simulink model "model_based_imp_ctrl_R2017a"  (Simulink 8.9)
settings: Solver=VariableStepAuto  StartTime=0.0  StopTime=20  FixedStep=0.00040  RelTol=1e-4  AbsTol=1e-7
InitFcn:
  | Parameter
values from neighbouring files (symbols this model uses):
  alpha = pi/180 * 13.6    (= 0.237364778271)    [IdealParameter.m]    (also in ParLuk11.m = deg2rad(13.6); Parameter.m = [-alpha_i;alpha_i;-alpha_i;alpha_i;-alpha_i;alpha_i]; ParameterIdeal.m = [-alpha_i;alpha_i;-alpha_i;alpha_i;-alpha_i;alpha_i]; ParameterVIVE.m = [alpha_i;-alpha_i;alpha_i;-alpha_i;alpha_i;-alpha_i])
  alpha_0 = alpha    (= 0.237364778271)    [IdealParameter.m]    (also in Parameter.m = alpha; ParameterIdeal.m = alpha*1.01; ParameterVIVE.m = alpha*1.01; ParameterVO.m = alpha*1.01)
  angular_noise = 0    [IdealParameter.m]    (also in Parameter.m = 0.5; ParameterIdeal.m; ParameterVIVE.m; ParameterVO.m)
  b = 1.1e-06    [IdealParameter.m]    (also in ParLuk11.m = 1.14e-07; Parameter.m; ParameterIdeal.m; ParameterVIVE.m)
  b_0 = b*1.15    (= 1.265e-06)    [IdealParameter.m]    (also in Parameter.m = 1.1e-06; ParameterIdeal.m; ParameterVIVE.m; ParameterVO.m)
  beta = 0    [IdealParameter.m]    (also in ParLuk11.m; Parameter.m = [beta_i; beta_i; beta_i; beta_i; beta_i; beta_i]; ParameterIdeal.m = [beta_i; beta_i; beta_i; beta_i; beta_i; beta_i]; ParameterVIVE.m = [beta_i; beta_i; beta_i; beta_i; beta_i; beta_i])
  beta_0 = beta    (= 0)    [IdealParameter.m]    (also in Parameter.m = beta; ParameterIdeal.m = beta*0.99; ParameterVIVE.m = beta*0.99; ParameterVO.m = beta*0.99)
  deltah = -0.0427    [Parameter.m]    (also in ParameterIdeal.m; ParameterVIVE.m = 0; ParameterVO.m; Parameter_old.m)
  deltah_0 = deltah    (= -0.0427)    [Parameter.m]    (also in ParameterIdeal.m = -0.041419; ParameterVIVE.m = 0; ParameterVO.m = -0.041419; Parameter_old.m = -0.041419)
  eta_rot = 50    [IdealParameter.m]    (also in Parameter.m = 2; ParameterIdeal.m = 20; ParameterVIVE.m = 5; ParameterVO.m = 2)
  g = 9.81    [IdealParameter.m]    (also in ParLuk11.m; Parameter.m; ParameterIdeal.m; ParameterVIVE.m)
  g_0 = g*0.99    (= 9.7119)    [IdealParameter.m]    (also in Parameter.m = 9.81; ParameterIdeal.m = 9.81; ParameterVIVE.m = 9.81; ParameterVO.m = 9.81)
  IB = [Ixx 0 0; 0 Iyy 0; 0 0 Izz]    [IdealParameter.m]    (also in ParLuk11.m; Parameter.m; ParameterIdeal.m; ParameterVIVE.m)
  IB_0 = IB*1.07    [IdealParameter.m]    (also in Parameter.m = IB; ParameterIdeal.m; ParameterVIVE.m; ParameterVO.m)
  Ip = [Ipx 0 0; 0 Ipy 0; 0 0 Ipz]    [Parameter.m]    (also in ParameterIdeal.m; ParameterVIVE.m; ParameterVO.m; Parameter_old.m)
  k = 5.6e-05    [IdealParameter.m]    (also in ParLuk11.m = 2.98e-06; Parameter.m; ParameterIdeal.m; ParameterVIVE.m = 5.13e-05)
  K_0 = Ts/(T_rotor_0+Ts)    (= 0.0384615384615)    [IdealParameter.m]    (also in Parameter.m = 0.230769230769; ParameterIdeal.m; ParameterVIVE.m = 0.0350877192982; ParameterVO.m = 0.214285714286)
  k_0 = k*1.16    (= 6.496e-05)    [IdealParameter.m]    (also in Parameter.m = 5.6e-05; ParameterIdeal.m; ParameterVIVE.m = 5.9508e-05; ParameterVO.m)
  K_d_star = 4*eye(3)    [Parameter.m]    (also in ParameterIdeal.m; ParameterVIVE.m; ParameterVO.m; Parameter_old.m)
  K_p_star = 50*eye(3)    [Parameter.m]    (also in ParameterIdeal.m; ParameterVIVE.m; ParameterVO.m; Parameter_old.m)
  L = 0.4    [IdealParameter.m]    (also in ParLuk11.m = 1; Parameter.m; ParameterIdeal.m; ParameterVIVE.m = 0.6)
  L_0 = L*1.02    (= 0.408)    [IdealParameter.m]    (also in Parameter.m = 0.4; ParameterIdeal.m; ParameterVIVE.m = 0.612; ParameterVO.m)
  lambda_rot = 10    [IdealParameter.m]    (also in Parameter.m = 3; ParameterIdeal.m; ParameterVIVE.m = 5; ParameterVO.m = 3)
  m = 1    [Controllability.m]    (also in IdealParameter.m = 2.5; ParLuk11.m = 0.6; Parameter.m = 4.85; ParameterIdeal.m = 4.85)
  m_0 = m*1.03    (= 2.575)    [IdealParameter.m]    (also in Parameter.m = 4.85; ParameterIdeal.m = 4.9955; ParameterVIVE.m = 4.52994; ParameterVO.m = 4.9955)
  M_rot = 50    [IdealParameter.m]    (also in Parameter.m = 6; ParameterIdeal.m = 15; ParameterVIVE.m = 1; ParameterVO.m = 6)
  M_star = m_0*eye(3)    [Parameter.m]    (also in ParameterIdeal.m; ParameterVIVE.m; ParameterVO.m; Parameter_old.m)
  mp = 0.05    [Parameter.m]    (also in ParameterIdeal.m; ParameterVIVE.m; ParameterVO.m; Parameter_old.m)
  omega_noise = 0    [IdealParameter.m]    (also in Parameter.m = sqrt(2)*angular_noise/Ts * pi/180; ParameterIdeal.m; ParameterVIVE.m; ParameterVO.m)
  p_noise = 0    [IdealParameter.m]    (also in Parameter.m = 0.001; ParameterIdeal.m; ParameterVIVE.m; ParameterVO.m)
  T_delay = 0    [IdealParameter.m]    (also in Parameter.m = 0.1; ParameterIdeal.m; ParameterVIVE.m = 0.04; ParameterVO.m = 0.1)
  T_rotor = 0.1    [IdealParameter.m]    (also in Parameter.m; ParameterIdeal.m; ParameterVIVE.m; ParameterVO.m)
  Ts = 1/250    (= 0.004)    [IdealParameter.m]    (also in Parameter.m = 0.03; ParameterIdeal.m; ParameterVIVE.m; ParameterVO.m = 0.03)
  v_noise = 0    [IdealParameter.m]    (also in Parameter.m = sqrt(2)*p_noise/Ts; ParameterIdeal.m; ParameterVIVE.m; ParameterVO.m)
  z_p_0 = T_rotor_0/(T_rotor_0+Ts)    (= 0.961538461538)    [IdealParameter.m]    (also in Parameter.m = 0.769230769231; ParameterIdeal.m; ParameterVIVE.m = 0.964912280702; ParameterVO.m = 0.785714285714)
undefined symbols (not defined in the file or in its folder): DiscIntNeverNeededParam, magnitude, mm
libraries: simulink x7, vrlib x2, slctrlblks x1, dspinverses x1
(part 1 of 3)
settings Model: Creator=jan  LastModifiedBy=chao
settings DataIOCC: LimitDataPoints=off  SaveFormat=Dataset  SignalLoggingSaveFormat=Dataset
settings DebuggingCC: UnderspecifiedInitializationDetection=Simplified  MergeDetectMultiDrivingBlocksExec=error  FcnCallInpInsideContextMsg=error  StateNameClashWarn=none  SFUnexpectedBacktrackingDiag=error  SFNoUnconditionalDefaultTransitionDiag=error
settings HardwareCC: ProdBitPerPointer=64  ProdBitPerSizeT=64  ProdBitPerPtrDiffT=64  ProdLargestAtomicFloat=Float  ProdIntDivRoundTo=Zero  ProdEndianess=LittleEndian  ProdWordSize=64  ProdHWDeviceType=Intel->x86-64 (Windows64)
settings ModelReferenceCC: PropagateSignalLabelsOutOfModel=on
settings GRTTargetCC: TargetLangStandard=C99 (ISO)  GeneratePreprocessorConditionals=Use local settings  CombineOutputUpdateFcns=on  GRTInterface=off
settings ConfigComp: CovMetricSettings=dwe  CovHtmlReporting=off  CovSaveCumulativeToWorkspaceVar=off  CovSaveSingleToWorkspaceVar=off  CovExternalEMLEnable=on

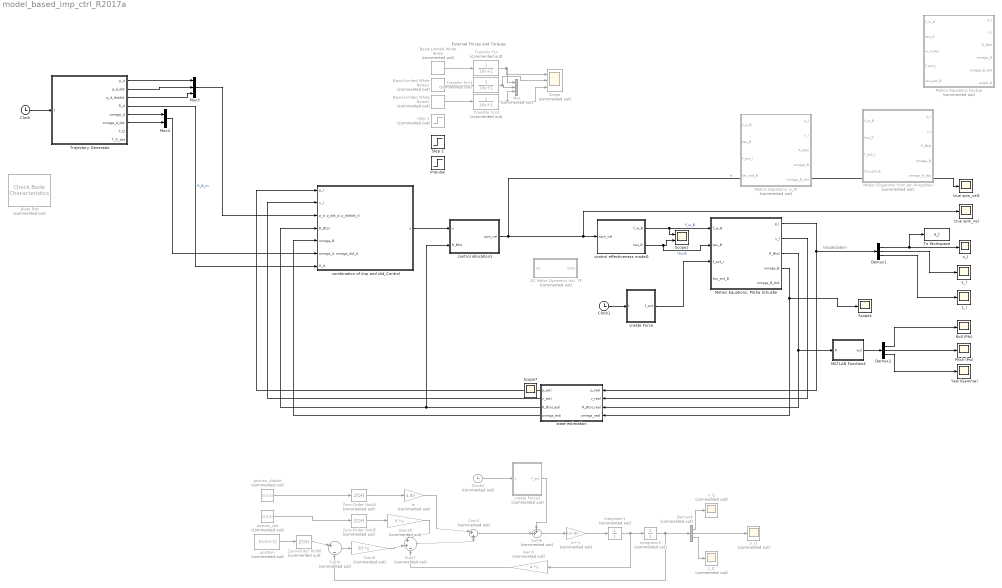
== system model_based_imp_ctrl_R2017a ==
  note: External Forces and Torques
  note: Visualization
  Band-Limited White Noise : simulink/Sources/Band-Limited White Noise  Commented=on  Cov=10  Ts=0.1  seed=[28341]  VectorParams1D=off
  Band-Limited White Noise1 : simulink/Sources/Band-Limited White Noise  Commented=on  Cov=10  Ts=0.1  seed=[23342]  VectorParams1D=off
  Band-Limited White Noise2 : simulink/Sources/Band-Limited White Noise  Commented=on  Cov=10  Ts=0.1  seed=[23441]  VectorParams1D=off
  Bode Plot : slctrlblks/Model Verification/Check Bode  Characteristics  Commented=on  InstantiateOnLoad=on  SaveOperatingPoints=off  LinearizationIOs={'/Trajectory Generator', 1, 'in', 'off', '';'/model3 Integral Sliding Mode Control', 1, 'out', 'off', ''}  LinearizeAt=SnapshotTimes  SnapshotTimes=[0]  TriggerType=rising  SampleTime=auto  RateConversionMethod=zoh  PreWarpFreq=10  UseExactDelayModel=off  UseFullBlockNameLabels=off  UseBusSignalLabels=off  enabled=on  stopWhenAssertionFail=off  export=off  ViewDlgPos=[100.333333333333 199.666666666667 510 390]  OpenViewOnLoad=off  LaunchViewOnOpen=off  FrequencyUnits=rad/s  MagnitudeUnits=dB  PhaseUnits=deg  TimeUnits=seconds  EnableUpperBound=off  UpperBoundFrequencies=[]  UpperBoundMagnitudes=[]  EnableLowerBound=off  LowerBoundFrequencies=[]  LowerBoundMagnitudes=[]
      settings: SourceProductName=Simulink Control Design
  Clock : Clock
  Clock1 : Clock
  Clock4 : Clock  Commented=on
  DC Motor Dynamics incl. FF : Subsystem  Commented=on  TreatAsAtomicUnit=on
  Demux1 : Demux  Outputs=3
  Demux2 : Demux  Outputs=3
  Demux4 : Demux  Commented=on  Outputs=3
  Gain10 : Gain  Commented=on  Gain=4  Multiplication=Matrix(K*u)
  Gain3 : Gain  Commented=on  Gain=4  Multiplication=Matrix(K*u)
  Gain9 : Gain  Commented=on  Gain=50  Multiplication=Matrix(K*u)
  Impulse : Step  Time=0.1  Before=[6,0,6]'  After=[0,0,0]'  SampleTime=0  VectorParams1D=off
  Integrator1 : Integrator  Commented=on  InitialCondition=[0 0 0]'
  Integrator2 : Integrator  Commented=on  InitialCondition=[0 0 0]'
  MATLAB Function4 : MATLAB Function  TreatAsAtomicUnit=on
  Motion Equations backup : Subsystem  Commented=on
  Motion Equations from Jan Krieglstein : Subsystem  Commented=on
  "Motion Equations, Micha Schuster" : Subsystem
  "Motion Equations, p_I3" : Subsystem  Commented=on
  Mux : Mux  Commented=on  Inputs=3
  Mux3 : Mux  Inputs=3
  Mux4 : Mux  Inputs=2
  Pitch (Psi) : Scope
  Roll (Phi) : Scope
  Scope : Scope  Commented=on  NumInputPorts=3
  Scope1 : Scope
  Scope2 : Scope  NumInputPorts=2
  Step 1 : Step  Commented=on  Before=[0;0;0]  After=[10;1;1]  SampleTime=0  VectorParams1D=off
  Step 2 : Step  Before=[0;0;0]  After=[5;1;1]  SampleTime=0  VectorParams1D=off
  Sum3 : Sum  Commented=on  Inputs=|+|+
  Sum6 : Sum  Commented=on  Inputs=++|
  Sum7 : Sum  Commented=on  Inputs=|+|+|-
  Sum8 : Sum  Commented=on  Inputs=|+|-
  To Workspace : ToWorkspace  VariableName=x_I  SaveFormat=Timeseries  SampleTime=-1
  Trajectory Generator : MATLAB Function  TreatAsAtomicUnit=on
  Transfer Fcn : TransferFcn  Commented=on  Denominator=[10 1]
  Transfer Fcn1 : TransferFcn  Commented=on  Denominator=[10 1]
  Transfer Fcn2 : TransferFcn  Commented=on  Denominator=[10 1]
  Yaw (Gamma) : Scope
  Zero-Order Hold4 : ZeroOrderHold  Commented=on  SampleTime=Ts
  Zero-Order Hold5 : ZeroOrderHold  Commented=on  SampleTime=Ts
  Zero-Order Hold6 : ZeroOrderHold  Commented=on  SampleTime=Ts
  combination of Imp and slid_Control : Subsystem
  control allocation1 : Subsystem
  control effectiveness model1 : Subsystem
  create Force : MATLAB Function  TreatAsAtomicUnit=on
  create Force2 : MATLAB Function  Commented=on  TreatAsAtomicUnit=on
  m : Gain  Commented=on  Gain=4.85
  m*-1 : Gain  Commented=on  Gain=1/4.85
  position : Constant  Commented=on  Value=[0;0;0.5]
  postion_dot : Constant  Commented=on  Value=[0;0;0]
  postion_dotdot : Constant  Commented=on  Value=[0;0;0]
  state estimation : Subsystem
  true spin_vel : Scope
  true spin_vel1 : Scope
  x_I : Scope
  x_I1 : Scope  Commented=on
  y_I : Scope
  y_I1 : Scope  Commented=on
  z_I : Scope
  z_I1 : Scope  Commented=on
  Scope7 : Scope
  wires:
  Demux2/2 -> Pitch (Psi)/1
  Demux1/3 -> z_I/1
  control allocation1/1(spin_vel) -> control effectiveness model1/1(spin_vel), true spin_vel/1, true spin_vel1/1  "u"
  Demux1/2 -> y_I/1
  Demux2/1 -> Roll (Phi)/1
  "Motion Equations, Micha Schuster"/3(R_BtoI) -> MATLAB Function4/1(R), state estimation/3(R_BtoI_real)
  Clock/1 -> Trajectory Generator/1(t)
  Trajectory Generator/3(p_d_dotdot) -> Mux3/3
  Trajectory Generator/2(p_d_dot) -> Mux3/2
  Trajectory Generator/6(omega_d_dot) -> Mux4/2
  Band-Limited White Noise/1 -> Transfer Fcn/1
  Transfer Fcn/1 -> Scope/1, Mux/1
  Transfer Fcn2/1 -> Scope/3, Mux/3
  Band-Limited White Noise1/1 -> Transfer Fcn1/1
  Band-Limited White Noise2/1 -> Transfer Fcn2/1
  Transfer Fcn1/1 -> Scope/2, Mux/2
  Trajectory Generator/5(omega_d) -> Mux4/1
  Demux2/3 -> Yaw (Gamma)/1
  MATLAB Function4/1(eul) -> Demux2/1
  "Motion Equations, Micha Schuster"/1(p_I) -> state estimation/1(p_real), Demux1/1
  Trajectory Generator/4(R_d) -> combination of Imp and slid_Control/7(R_d)  "R_B_m"
  Mux3/1 -> combination of Imp and slid_Control/3("p_d, p_dot_d, p_dotdot_d")
  Mux4/1 -> combination of Imp and slid_Control/6("omega_d, omega_dot_d")
  Clock1/1 -> create Force/1(t)
  Trajectory Generator/1(p_d) -> Mux3/1
  Gain10/1 -> Sum7/1
  Zero-Order Hold6/1 -> Sum8/1
  Integrator2/1 -> Demux4/1, Sum8/2
  m*-1/1 -> Integrator1/1
  Demux4/1 -> x_I1/1
  Sum7/1 -> Sum3/2
  postion_dot/1 -> Zero-Order Hold5/1
  Demux4/2 -> y_I1/1
  Zero-Order Hold4/1 -> m/1
  Sum6/1 -> m*-1/1
  Integrator1/1 -> Gain3/1, Integrator2/1
  position/1 -> Zero-Order Hold6/1
  Zero-Order Hold5/1 -> Gain10/1
  m/1 -> Sum3/1
  Sum3/1 -> Sum6/2
  Demux4/3 -> z_I1/1
  Gain9/1 -> Sum7/2
  Gain3/1 -> Sum7/3
  postion_dotdot/1 -> Zero-Order Hold4/1
  Sum8/1 -> Gain9/1
  create Force2/1(f_ext) -> Sum6/1
  Clock4/1 -> create Force2/1(t)
  combination of Imp and slid_Control/1(u) -> control allocation1/1(u)
  state estimation/3(R_BtoI_esti) -> control allocation1/2(R_BtoI), combination of Imp and slid_Control/4(R_BtoI)
  state estimation/4(omega_esti) -> combination of Imp and slid_Control/5(omega_B)
  state estimation/2(v_esti) -> combination of Imp and slid_Control/2(v_I)
  state estimation/1(p_esti) -> combination of Imp and slid_Control/1(p_I)
  "Motion Equations, Micha Schuster"/2(v_I) -> state estimation/2(v_real)
  "Motion Equations, Micha Schuster"/4(omega_B) -> Scope1/1, state estimation/4(omega_real)
  control effectiveness model1/1(f_w_B) -> "Motion Equations, Micha Schuster"/1("f_w_B "), Scope2/1  "f_w_B"
  control effectiveness model1/2(tau_B) -> "Motion Equations, Micha Schuster"/2(tau_B), Scope2/2  "tau_B"
  create Force/1(f_ext) -> "Motion Equations, Micha Schuster"/3(f_ext_I)
  Demux1/1 -> To Workspace/1, x_I/1

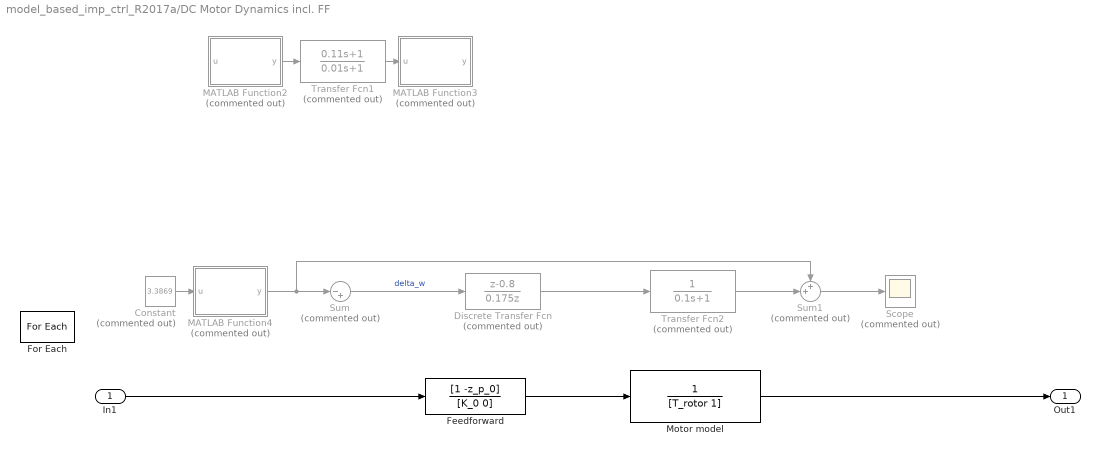
== system model_based_imp_ctrl_R2017a/DC Motor Dynamics incl. FF ==
  In1 : Inport  Partition=on  PartitionDimension=1  PartitionWidth=1
  Constant : Constant  Commented=on  Value=3.3869
  Discrete Transfer Fcn : DiscreteTransferFcn  Commented=on  Numerator=[1 -0.8]  Denominator=[0.175 0]  SampleTime=Ts
  Feedforward : DiscreteTransferFcn  Numerator=[1 -z_p_0]  Denominator=[K_0 0]  InitialStates=274  SampleTime=Ts
  For Each : ForEach  DisableCoverage=on  IndexMode=One-based
  MATLAB Function2 : MATLAB Function  Commented=on  TreatAsAtomicUnit=on
  MATLAB Function3 : MATLAB Function  Commented=on  TreatAsAtomicUnit=on
  MATLAB Function4 : MATLAB Function  Commented=on  TreatAsAtomicUnit=on
  Motor model : TransferFcn  Denominator=[T_rotor 1]
  Scope : Scope  Commented=on
  Sum : Sum  Commented=on  Inputs=|-+
  Sum1 : Sum  Commented=on  Inputs=++|
  Transfer Fcn1 : TransferFcn  Commented=on  Numerator=[0.11 1]  Denominator=[0.01 1]
  Transfer Fcn2 : TransferFcn  Commented=on  Denominator=[0.1 1]
  Out1 : Outport  ConcatenationDimension=1
  wires:
  Transfer Fcn1/1 -> MATLAB Function3/1(u)
  MATLAB Function2/1(y) -> Transfer Fcn1/1
  Constant/1 -> MATLAB Function4/1(u)
  MATLAB Function4/1(y) -> Sum1/1, Sum/1
  Sum/1 -> Discrete Transfer Fcn/1  "delta_w"
  In1/1 -> Feedforward/1
  Discrete Transfer Fcn/1 -> Transfer Fcn2/1
  Transfer Fcn2/1 -> Sum1/2
  Motor model/1 -> Out1/1
  Sum1/1 -> Scope/1
  Feedforward/1 -> Motor model/1

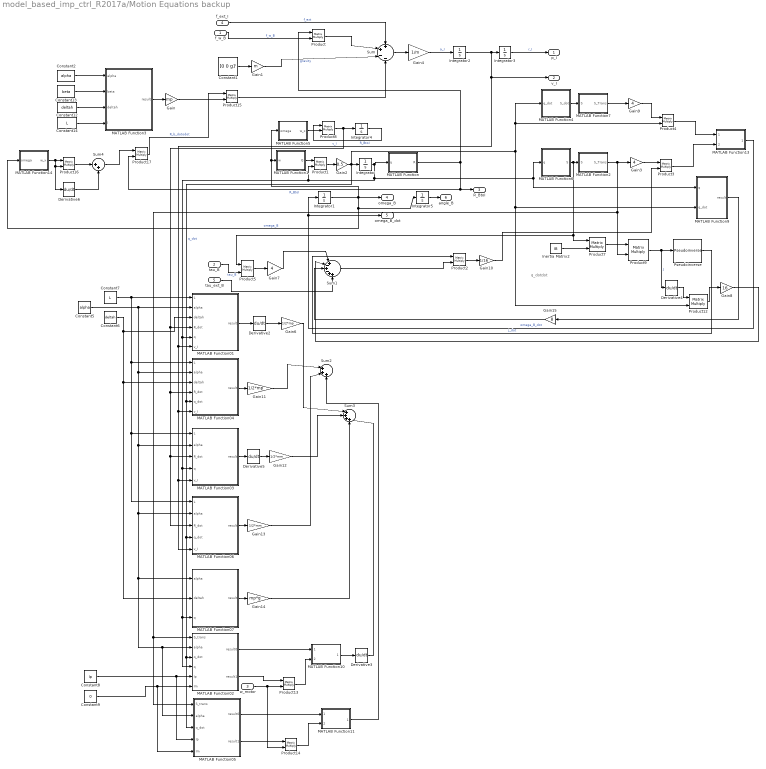
== system model_based_imp_ctrl_R2017a/Motion Equations backup ==
  note: q_dotdot
  "f_w_B " : Inport
  tau_B : Inport  Port=2
  w_motor : Inport  Port=3
  f_ext_I : Inport  Port=4
  tau_ext_B : Inport  Port=5
  Constant1 : Constant  Value=[0 0 g]'  VectorParams1D=off
  Constant12 : Constant  Value=deltah
  Constant13 : Constant  Value=beta
  Constant14 : Constant  Value=L
  Constant2 : Constant  Value=alpha
  Constant5 : Constant  Value=alpha
  Constant6 : Constant  Value=deltah
  Constant7 : Constant  Value=L
  Constant8 : Constant  Value=Ip
  Constant9 : Constant  Value=0
  Derivative{2..6} (5 alike) : Derivative  CoefficientInTFapproximation=0
  Gain : Gain  Gain=mp
  Gain1 : Gain  Gain=m
  Gain10 : Gain  Gain=1/16
  Gain11 : Gain  Gain=1/2*mp
  Gain12 : Gain  Gain=1/2*mm
  Gain13 : Gain  Gain=1/2*mm
  Gain14 : Gain  Gain=mp*g
  Gain15 : Gain  Gain=8
  Gain2 : Gain  Gain=0.5
  Gain3 : Gain  Gain=4
  Gain4 : Gain  Gain=1/m
  Gain6 : Gain  Gain=1/2*mp
  Gain7 : Gain  Gain=4
  Gain8 : Gain  Gain=16
  Gain9 : Gain  Gain=4
  Inertia Matrix2 : Constant  Value=IB  VectorParams1D=off
  Integrator : Integrator  InitialCondition=[0 0 0 1]
  Integrator1 : Integrator  InitialCondition=[0 0 0]'
  Integrator2 : Integrator  InitialCondition=[0;0;0]
  Integrator3 : Integrator  InitialCondition=[0 0 0]'
  Integrator4 : Integrator  InitialCondition=[1 0 0; 0 1 0; 0 0 1]
  Integrator5 : Integrator  InitialCondition=[0 0 0]'
  MATLAB Function : MATLAB Function  TreatAsAtomicUnit=on
  MATLAB Function01 : MATLAB Function  TreatAsAtomicUnit=on
  MATLAB Function02 : MATLAB Function  TreatAsAtomicUnit=on
  MATLAB Function03 : MATLAB Function  TreatAsAtomicUnit=on
  MATLAB Function04 : MATLAB Function  TreatAsAtomicUnit=on
  MATLAB Function05 : MATLAB Function  TreatAsAtomicUnit=on
  MATLAB Function06 : MATLAB Function  TreatAsAtomicUnit=on
  MATLAB Function07 : MATLAB Function  TreatAsAtomicUnit=on
  MATLAB Function1 : MATLAB Function  TreatAsAtomicUnit=on
  MATLAB Function10 : MATLAB Function  TreatAsAtomicUnit=on
  MATLAB Function11 : MATLAB Function  TreatAsAtomicUnit=on
  MATLAB Function13 : MATLAB Function  TreatAsAtomicUnit=on
  MATLAB Function14 : MATLAB Function  TreatAsAtomicUnit=on
  MATLAB Function2 : MATLAB Function  TreatAsAtomicUnit=on
  MATLAB Function3 : MATLAB Function  TreatAsAtomicUnit=on
  MATLAB Function4 : MATLAB Function  TreatAsAtomicUnit=on
  MATLAB Function5 : MATLAB Function  TreatAsAtomicUnit=on
  MATLAB Function6 : MATLAB Function  TreatAsAtomicUnit=on
  MATLAB Function7 : MATLAB Function  TreatAsAtomicUnit=on
  MATLAB Function9 : MATLAB Function  TreatAsAtomicUnit=on
  Product{,1..5,7..9,12..17} (15 alike) : Product  Multiplication=Matrix(*)
  Pseudoinverse : dspinverses/Pseudoinverse  wanterr=off  SimulateUsing=Interpreted execution
      settings: SourceProductName=DSP System Toolbox  SourceProductBaseCode=DS
  Sum : Sum  Inputs=++--
  Sum1 : Sum  Inputs=|+-+-++
  Sum2 : Sum  Inputs=|+++
  Sum3 : Sum  Inputs=|++++
  Sum4 : Sum  Inputs=|++
  p_I : Outport
  v_I : Outport  Port=2
  R_BtoI : Outport  Port=3
  omega_B : Outport  Port=4
  omega_B_dot : Outport  Port=5
  angle_B : Outport  Port=6
  wires:
  Gain4/1 -> Integrator2/1  "a_I"
  Constant1/1 -> Gain1/1
  Gain2/1 -> MATLAB Function04/5(q_dot), MATLAB Function06/4(q_dot), MATLAB Function05/3(q_dot), MATLAB Function02/3(q_dot), MATLAB Function4/1(q_dot), Product4/2, MATLAB Function9/2(q_dot), Product12/2, Integrator/1  "q_dot"
  Integrator2/1 -> MATLAB Function06/5(v_I), MATLAB Function03/5(v_I), MATLAB Function04/6(v_I), MATLAB Function01/6(v_I), v_I/1, Integrator3/1  "v_I"
  Sum/1 -> Gain4/1
  "f_w_B "/1 -> Product/2  "f_w_B"
  Product1/1 -> Gain2/1
  Integrator3/1 -> p_I/1  "r_I"
  MATLAB Function1/1(Q) -> Product1/1
  MATLAB Function/1(R) -> Product/1, Product17/2, R_BtoI/1  "R_BtoI"
  tau_B/1 -> Product5/2  "tau_B"
  Sum1/1 -> Product2/2
  MATLAB Function4/1(S_dot) -> MATLAB Function7/1(S)
  MATLAB Function7/1(S_Trans) -> Gain9/1
  Gain3/1 -> Product3/1
  Gain9/1 -> Product4/1
  Product4/1 -> MATLAB Function13/1(factor1)
  Product3/1 -> MATLAB Function13/2(factor2)
  MATLAB Function13/1(add_result) -> Integrator1/1, omega_B_dot/1  "omega_B_dot"
  MATLAB Function6/1(S) -> Product5/1, Product7/1, MATLAB Function2/1(S)
  Product5/1 -> Gain7/1
  Gain7/1 -> Sum1/1
  Inertia Matrix2/1 -> Product7/2
  Product7/1 -> Product9/1
  Product9/1 -> Derivative4/1, Pseudoinverse/1  "J"
  Pseudoinverse/1 -> Product2/1  "j_dot"
  Derivative4/1 -> Product12/1
  Product8/1 -> MATLAB Function06/3(R_dot), MATLAB Function03/3(R_dot), MATLAB Function04/4(R_dot), MATLAB Function01/4(R_dot), Integrator4/1
  Integrator4/1 -> Product8/1  "R_BtoI"
  MATLAB Function5/1(w_x) -> Product8/2
  Integrator1/1 -> MATLAB Function14/1(omega), Integrator5/1, MATLAB Function5/1(omega), MATLAB Function1/1(w), omega_B/1  "omega_B"
  Derivative2/1 -> Gain6/1
  MATLAB Function01/1(result) -> Derivative2/1
  Constant6/1 -> MATLAB Function07/2(deltah), MATLAB Function04/3(deltah), MATLAB Function01/3(deltah)
  Constant5/1 -> MATLAB Function03/2(alpha), MATLAB Function06/2(alpha), MATLAB Function07/1(alpha), MATLAB Function05/2(alpha), MATLAB Function02/2(alpha), MATLAB Function04/2(alpha), MATLAB Function01/2(alpha)
  Product12/1 -> Gain8/1
  Gain8/1 -> Sum1/2
  Product2/1 -> Gain10/1
  Gain10/1 -> Product3/2
  Integrator/1 -> MATLAB Function03/4(q), MATLAB Function07/3(q), MATLAB Function02/4(q), MATLAB Function01/5(q), Product1/2, MATLAB Function6/1(q), MATLAB Function9/1(q), MATLAB Function/1(q)
  Constant7/1 -> MATLAB Function06/1(L), MATLAB Function03/1(L), MATLAB Function04/1(L), MATLAB Function01/1(L)
  MATLAB Function04/1(result) -> Gain11/1
  MATLAB Function2/1(S_Trans) -> MATLAB Function05/1(S_trans), MATLAB Function02/1(S_trans), Product9/2, Gain3/1
  Constant8/1 -> MATLAB Function05/4(Ip), MATLAB Function02/5(Ip)
  Constant9/1 -> MATLAB Function05/5(Im), MATLAB Function02/6(Im)
  MATLAB Function03/1(result) -> Derivative5/1
  Derivative5/1 -> Gain12/1
  MATLAB Function06/1(result) -> Gain13/1
  MATLAB Function07/1(result) -> Gain14/1
  Gain6/1 -> Sum3/1
  Gain11/1 -> Sum2/1
  Gain12/1 -> Sum3/2
  Gain13/1 -> Sum2/2
  MATLAB Function02/2(result1) -> Product13/1
  MATLAB Function02/1(result0) -> MATLAB Function10/1(factor1)
  Product13/1 -> MATLAB Function10/2(factor2)
  MATLAB Function10/1(add_result) -> Derivative3/1
  Gain14/1 -> Sum3/4
  Derivative3/1 -> Sum3/3
  w_motor/1 -> Product14/2, Product13/2
  MATLAB Function05/2(result1) -> Product14/1
  MATLAB Function05/1(result0) -> MATLAB Function11/1(factor1)
  Product14/1 -> MATLAB Function11/2(factor2)
  MATLAB Function11/1(add_result) -> Sum2/3
  MATLAB Function9/1(result) -> Gain15/1
  Gain15/1 -> Sum1/3
  f_ext_I/1 -> Sum/1  "f_ext"
  Product/1 -> Sum/2
  Gain1/1 -> Sum/3  "gravity"
  tau_ext_B/1 -> Sum1/6
  Integrator5/1 -> angle_B/1
  Product17/1 -> Product15/1  "R_b_dotodot"
  Product15/1 -> Sum/4
  MATLAB Function14/1(w_x) -> Derivative6/1, Product16/2, Product16/1
  Product16/1 -> Sum4/1
  Derivative6/1 -> Sum4/2
  Sum4/1 -> Product17/1
  Constant13/1 -> MATLAB Function3/2(beta)
  Constant2/1 -> MATLAB Function3/1(alpha)
  Constant12/1 -> MATLAB Function3/3(deltah)
  MATLAB Function3/1(result) -> Gain/1
  Constant14/1 -> MATLAB Function3/4(l)
  Gain/1 -> Product15/2

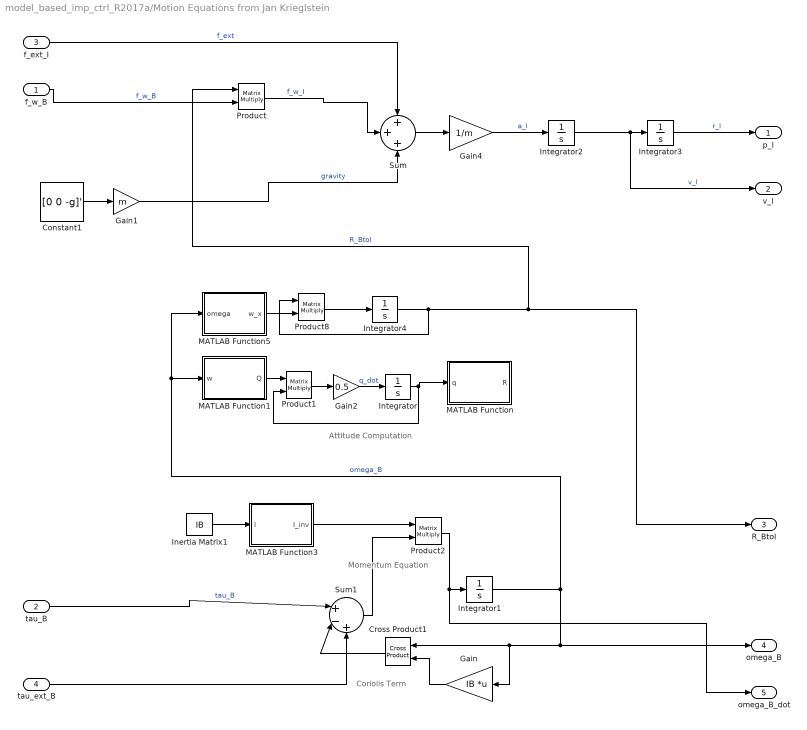
== system model_based_imp_ctrl_R2017a/Motion Equations from Jan Krieglstein ==
  note: Momentum Equation
  note: Attitude Computation
  note: Coriolis Term
  "f_w_B " : Inport
  tau_B : Inport  Port=2
  f_ext_I : Inport  Port=3
  tau_ext_B : Inport  Port=4
  Constant1 : Constant  Value=[0 0 -g]'  VectorParams1D=off
  Cross Product1 : vrlib/Utilities/Cross Product
      settings: SourceProductBaseCode=VR
  Gain : Gain  Gain=IB  Multiplication=Matrix(K*u)
  Gain1 : Gain  Gain=m
  Gain2 : Gain  Gain=0.5
  Gain4 : Gain  Gain=1/m
  Inertia Matrix1 : Constant  Value=IB  VectorParams1D=off
  Integrator : Integrator  InitialCondition=[0 0 0 1]
  Integrator1 : Integrator  InitialCondition=[0 0 0]'
  Integrator2 : Integrator  InitialCondition=[0;0;0]
  Integrator3 : Integrator  InitialCondition=[0 0 0]'
  Integrator4 : Integrator  InitialCondition=[1 0 0; 0 1 0; 0 0 1]
  MATLAB Function : MATLAB Function  TreatAsAtomicUnit=on
  MATLAB Function1 : MATLAB Function  TreatAsAtomicUnit=on
  MATLAB Function3 : MATLAB Function  TreatAsAtomicUnit=on
  MATLAB Function5 : MATLAB Function  TreatAsAtomicUnit=on
  Product{,1..2,8} (4 alike) : Product  Multiplication=Matrix(*)
  Sum : Sum  Inputs=+++
  Sum1 : Sum  Inputs=|+-+
  p_I : Outport
  v_I : Outport  Port=2
  R_BtoI : Outport  Port=3
  omega_B : Outport  Port=4
  omega_B_dot : Outport  Port=5
  wires:
  Product2/1 -> omega_B_dot/1, Integrator1/1
  Gain/1 -> Cross Product1/2
  Gain4/1 -> Integrator2/1  "a_I"
  Constant1/1 -> Gain1/1
  Gain2/1 -> Integrator/1  "q_dot"
  Integrator2/1 -> v_I/1, Integrator3/1  "v_I"
  tau_B/1 -> Sum1/1  "tau_B"
  Integrator/1 -> Product1/2, MATLAB Function/1(q)
  Sum1/1 -> Product2/2
  Sum/1 -> Gain4/1
  "f_w_B "/1 -> Product/2  "f_w_B"
  Product1/1 -> Gain2/1
  Gain1/1 -> Sum/3  "gravity"
  Cross Product1/1 -> Sum1/2
  Integrator3/1 -> p_I/1  "r_I"
  MATLAB Function1/1(Q) -> Product1/1
  Integrator1/1 -> omega_B/1, Gain/1, Cross Product1/1, MATLAB Function5/1(omega), MATLAB Function1/1(w)  "omega_B"
  Product/1 -> Sum/2  "f_w_I"
  MATLAB Function5/1(w_x) -> Product8/2
  Product8/1 -> Integrator4/1
  Integrator4/1 -> Product8/1, Product/1, R_BtoI/1  "R_BtoI"
  f_ext_I/1 -> Sum/1  "f_ext"
  tau_ext_B/1 -> Sum1/3
  MATLAB Function3/1(I_inv) -> Product2/1
  Inertia Matrix1/1 -> MATLAB Function3/1(I)

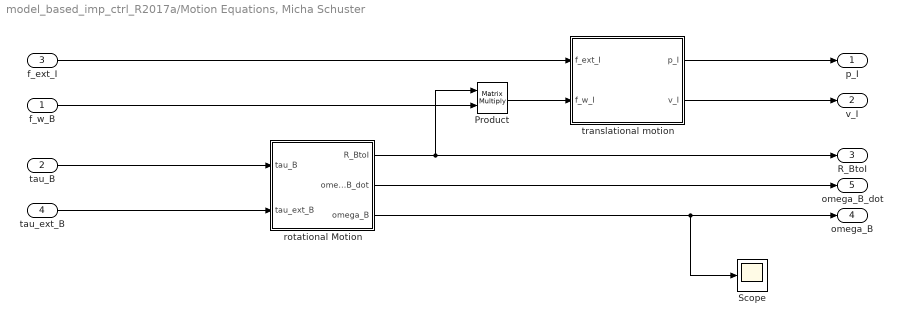
== system model_based_imp_ctrl_R2017a/Motion Equations, Micha Schuster ==
  "f_w_B " : Inport
  tau_B : Inport  Port=2
  f_ext_I : Inport  Port=3
  tau_ext_B : Inport  Port=4
  Product : Product  Multiplication=Matrix(*)
  Scope : Scope
  rotational Motion : Subsystem
  translational motion : Subsystem
  p_I : Outport
  v_I : Outport  Port=2
  R_BtoI : Outport  Port=3
  omega_B : Outport  Port=4
  omega_B_dot : Outport  Port=5
  wires:
  f_ext_I/1 -> translational motion/1(f_ext_I)
  translational motion/1(p_I) -> p_I/1
  translational motion/2(v_I) -> v_I/1
  Product/1 -> translational motion/2(f_w_I)
  rotational Motion/1(R_BtoI) -> Product/1, R_BtoI/1
  tau_B/1 -> rotational Motion/1(tau_B)
  tau_ext_B/1 -> rotational Motion/2(tau_ext_B)
  rotational Motion/2(omega_B_dot) -> omega_B_dot/1
  rotational Motion/3(omega_B) -> Scope/1, omega_B/1
  "f_w_B "/1 -> Product/2

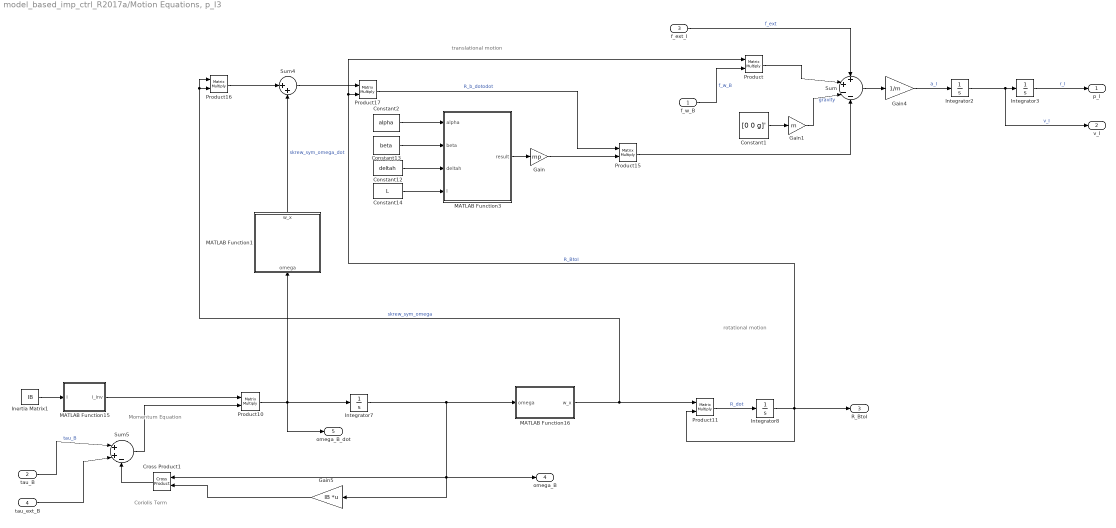
== system model_based_imp_ctrl_R2017a/Motion Equations, p_I3 ==
  note: Coriolis Term
  note: rotational motion
  note: Momentum Equation
  note: translational motion
  "f_w_B " : Inport
  tau_B : Inport  Port=2
  f_ext_I : Inport  Port=3
  tau_ext_B : Inport  Port=4
  Constant1 : Constant  Value=[0 0 g]'  VectorParams1D=off
  Constant12 : Constant  Value=deltah
  Constant13 : Constant  Value=beta
  Constant14 : Constant  Value=L
  Constant2 : Constant  Value=alpha
  Cross Product1 : vrlib/Utilities/Cross Product
      settings: SourceProductBaseCode=VR
  Gain : Gain  Gain=mp
  Gain1 : Gain  Gain=m
  Gain4 : Gain  Gain=1/m
  Gain5 : Gain  Gain=IB  Multiplication=Matrix(K*u)
  Inertia Matrix1 : Constant  Value=IB  VectorParams1D=off
  Integrator2 : Integrator  InitialCondition=[0;0;0]
  Integrator3 : Integrator  InitialCondition=[0 0 0]'
  Integrator7 : Integrator  InitialCondition=[0 0 0]'
  Integrator8 : Integrator  InitialCondition=[1 0 0; 0 1 0; 0 0 1]
  MATLAB Function1 : MATLAB Function  TreatAsAtomicUnit=on
  MATLAB Function15 : MATLAB Function  TreatAsAtomicUnit=on
  MATLAB Function16 : MATLAB Function  TreatAsAtomicUnit=on
  MATLAB Function3 : MATLAB Function  TreatAsAtomicUnit=on
  Product{,10..11,15..17} (6 alike) : Product  Multiplication=Matrix(*)
  Sum : Sum  Inputs=++--
  Sum4 : Sum  Inputs=|++
  Sum5 : Sum  Inputs=|++-
  p_I : Outport
  v_I : Outport  Port=2
  R_BtoI : Outport  Port=3
  omega_B : Outport  Port=4
  omega_B_dot : Outport  Port=5
  wires:
  Gain4/1 -> Integrator2/1  "a_I"
  Constant1/1 -> Gain1/1
  Integrator2/1 -> v_I/1, Integrator3/1  "v_I"
  Sum/1 -> Gain4/1
  "f_w_B "/1 -> Product/2  "f_w_B"
  Integrator3/1 -> p_I/1  "r_I"
  f_ext_I/1 -> Sum/1  "f_ext"
  Product/1 -> Sum/2
  Gain1/1 -> Sum/3  "gravity"
  Product17/1 -> Product15/1  "R_b_dotodot"
  Product15/1 -> Sum/4
  MATLAB Function16/1(w_x) -> Product11/1, Product16/1, Product16/2  "skrew_sym_omega"
  Product16/1 -> Sum4/1
  Product10/1 -> Integrator7/1, omega_B_dot/1, MATLAB Function1/1(omega)
  Sum4/1 -> Product17/1
  Constant13/1 -> MATLAB Function3/2(beta)
  Constant2/1 -> MATLAB Function3/1(alpha)
  Constant12/1 -> MATLAB Function3/3(deltah)
  MATLAB Function3/1(result) -> Gain/1
  Constant14/1 -> MATLAB Function3/4(l)
  Gain/1 -> Product15/2
  tau_ext_B/1 -> Sum5/2
  tau_B/1 -> Sum5/1  "tau_B"
  Inertia Matrix1/1 -> MATLAB Function15/1(I)
  Integrator7/1 -> Cross Product1/1, Gain5/1, omega_B/1, MATLAB Function16/1(omega)
  Gain5/1 -> Cross Product1/2
  Cross Product1/1 -> Sum5/3
  Product11/1 -> Integrator8/1  "R_dot"
  MATLAB Function15/1(I_inv) -> Product10/1
  Integrator8/1 -> Product/1, Product17/2, R_BtoI/1, Product11/2  "R_BtoI"
  Sum5/1 -> Product10/2
  MATLAB Function1/1(w_x) -> Sum4/2  "skrew_sym_omega_dot"

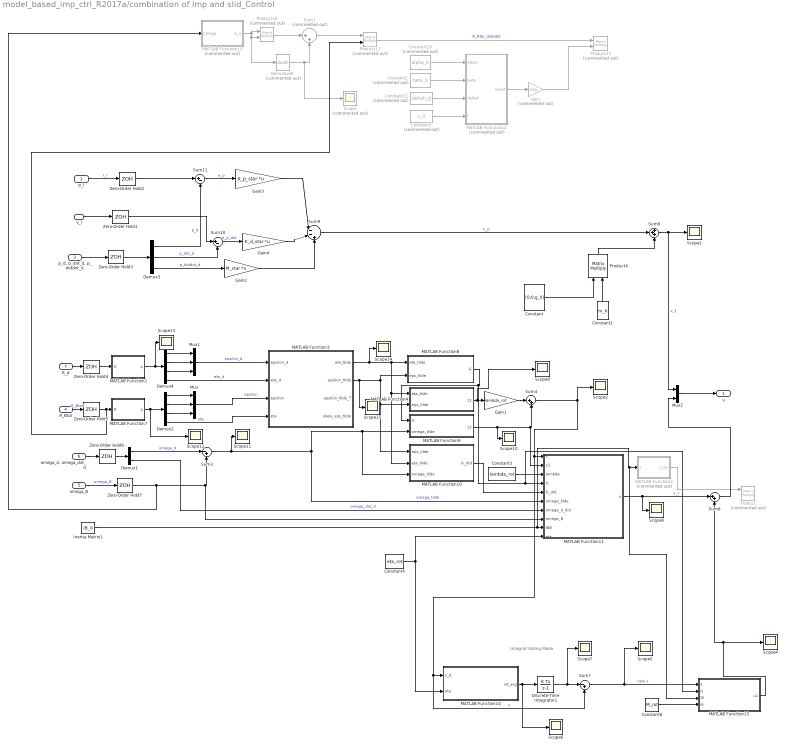
== system model_based_imp_ctrl_R2017a/combination of Imp and slid_Control ==
  note: Integral Sliding Mode
  p_I : Inport
  v_I : Inport  Port=2
  "p_d, p_dot_d, p_dotdot_d" : Inport  Port=3
  R_BtoI : Inport  Port=4
  omega_B : Inport  Port=5
  "omega_d, omega_dot_d" : Inport  Port=6
  R_d : Inport  Port=7
  Constant : Constant  Value=[0;0;g_0]  VectorParams1D=off
  Constant1 : Constant  Value=m_0
  Constant10 : Constant  Commented=on  Value=alpha_0
  Constant11 : Constant  Commented=on  Value=deltah_0
  Constant2 : Constant  Commented=on  Value=beta_0
  Constant3 : Constant  Value=lambda_rot
  Constant4 : Constant  Value=eta_rot
  Constant5 : Constant  Commented=on  Value=L_0
  Constant6 : Constant  Value=M_rot
  Demux1 : Demux  Outputs=2
  Demux2 : Demux
  Demux3 : Demux  Outputs=3
  Demux4 : Demux
  Derivative6 : Derivative  Commented=on  CoefficientInTFapproximation=0
  Discrete-Time Integrator1 : DiscreteIntegrator  InitialCondition=[0;0;0;0]  InitialConditionSetting=State (most efficient)  SampleTime=Ts  ICPrevOutput=DiscIntNeverNeededParam  ICPrevScaledInput=DiscIntNeverNeededParam
  Gain : Gain  Commented=on  Gain=mp
  Gain1 : Gain  Gain=lambda_rot
  Gain2 : Gain  Gain=M_star  Multiplication=Matrix(K*u)
  Gain3 : Gain  Gain=K_p_star  Multiplication=Matrix(K*u)
  Gain4 : Gain  Gain=K_d_star  Multiplication=Matrix(K*u)
  Inertia Matrix1 : Constant  Value=IB_0  VectorParams1D=off
  MATLAB Function1 : MATLAB Function  TreatAsAtomicUnit=on
  MATLAB Function10 : MATLAB Function  TreatAsAtomicUnit=on  SystemSampleTime=Ts
  MATLAB Function11 : MATLAB Function  TreatAsAtomicUnit=on  SystemSampleTime=Ts
  MATLAB Function12 : MATLAB Function  Commented=on  TreatAsAtomicUnit=on
  MATLAB Function13 : MATLAB Function  Commented=on  TreatAsAtomicUnit=on
  MATLAB Function14 : MATLAB Function  TreatAsAtomicUnit=on  SystemSampleTime=Ts
  MATLAB Function15 : MATLAB Function  TreatAsAtomicUnit=on  SystemSampleTime=Ts
  MATLAB Function2 : MATLAB Function  Commented=on  TreatAsAtomicUnit=on  SystemSampleTime=Ts
  MATLAB Function3 : MATLAB Function  TreatAsAtomicUnit=on  SystemSampleTime=Ts
  MATLAB Function4 : MATLAB Function  TreatAsAtomicUnit=on  SystemSampleTime=Ts
  MATLAB Function7 : MATLAB Function  TreatAsAtomicUnit=on
  MATLAB Function8 : MATLAB Function  TreatAsAtomicUnit=on  SystemSampleTime=Ts
  MATLAB Function9 : MATLAB Function  TreatAsAtomicUnit=on  SystemSampleTime=Ts
  Mux : Mux  Inputs=3
  Mux1 : Mux  Inputs=3
  Mux2 : Mux  Inputs=2
  Product{,15..17} (4 alike) : Product  Commented=on  Multiplication=Matrix(*)
  Product4 : Product  Inputs=**  Multiplication=Matrix(*)
  Scope : Scope  Commented=on
  Scope{1..2,4..15} (14 alike) : Scope
  Sum1 : Sum  Commented=on  Inputs=|++
  Sum10 : Sum  Inputs=|+-
  Sum11 : Sum  Inputs=|+-
  Sum3 : Sum  Inputs=|-+
  Sum4 : Sum  Inputs=|++
  Sum6 : Sum  Inputs=+++
  Sum7 : Sum  Inputs=|-+
  Sum8 : Sum  Inputs=|++
  Sum9 : Sum  Inputs=|--+
  Zero-Order Hold{1..7} (7 alike) : ZeroOrderHold  SampleTime=Ts
  u : Outport
  wires:
  Sum6/1 -> Mux2/1, Scope1/1  "v_t"
  Demux1/1 -> Sum3/1  "omega_d"
  Inertia Matrix1/1 -> MATLAB Function11/9(IBB), MATLAB Function15/3(IB), MATLAB Function2/1(I)
  Demux1/2 -> MATLAB Function11/7(omega_d_dot)  "omega_dot_d"
  Demux4/2 -> Mux1/2
  Demux2/4 -> MATLAB Function3/4(eta)  "eta"
  Demux2/1 -> Mux/1
  Mux1/1 -> MATLAB Function3/1(epsilon_d)  "epsilon_d"
  Demux4/1 -> Mux1/1
  MATLAB Function7/1(q) -> Scope12/1, Demux2/1
  Mux/1 -> MATLAB Function3/3(epsilon)  "epsilon"
  MATLAB Function1/1(q) -> Scope13/1, Demux4/1
  Demux2/2 -> Mux/2
  Demux2/3 -> Mux/3
  Demux4/3 -> Mux1/3
  Demux4/4 -> MATLAB Function3/2(eta_d)  "eta_d"
  MATLAB Function3/1(eta_tilde) -> Scope14/1, MATLAB Function10/2(eta_tilde), MATLAB Function4/1(eta_tilde), MATLAB Function8/1(eta_tilde)
  MATLAB Function8/1(G) -> MATLAB Function15/2(G), MATLAB Function11/4(G), MATLAB Function9/1(G)
  omega_B/1 -> Zero-Order Hold7/1  "omega_B"
  Sum3/1 -> Scope11/1, MATLAB Function11/6(omega_tilde), MATLAB Function10/3(omega_tilde), MATLAB Function9/2(omega_tilde)  "omega_tilde"
  MATLAB Function9/1(z2) -> Scope10/1, MATLAB Function11/2(z2), Sum4/2
  MATLAB Function4/1(z1) -> Scope9/1, Gain1/1
  Gain1/1 -> Sum4/1
  Constant4/1 -> MATLAB Function11/10(eta), MATLAB Function14/2(eta)
  Constant3/1 -> MATLAB Function11/3(lambda)
  MATLAB Function10/1(G_dot) -> MATLAB Function11/5(G_dot)
  Discrete-Time Integrator1/1 -> Scope7/1, Sum7/1
  Constant6/1 -> MATLAB Function15/4(M)
  Sum4/1 -> Scope2/1, MATLAB Function14/1(s_0), Sum7/2, MATLAB Function11/1(s)  "s"
  MATLAB Function14/1(int_arg) -> Scope6/1, Discrete-Time Integrator1/1
  Sum7/1 -> MATLAB Function15/1(s), Scope5/1  "new s"
  MATLAB Function2/1(I_inv) -> Product/1
  R_d/1 -> Zero-Order Hold4/1
  "omega_d, omega_dot_d"/1 -> Zero-Order Hold6/1
  MATLAB Function15/1(u1) -> Sum8/2, Scope4/1
  Sum8/1 -> Mux2/2
  MATLAB Function11/1(u) -> Scope8/1, Sum8/1  "v_r"
  MATLAB Function3/2(epsilon_tilde) -> Scope15/1, MATLAB Function10/1(eps_tilde), MATLAB Function4/2(eps_tilde), MATLAB Function8/2(eps_tilde)
  Demux3/2 -> Sum10/2  "p_dot_d"
  Demux3/1 -> Sum11/2  "p_d"
  p_I/1 -> Zero-Order Hold2/1  "r_I"
  Gain4/1 -> Sum9/2
  Sum10/1 -> Gain4/1  "e_p_dot"
  Sum11/1 -> Gain3/1  "e_p"
  Demux3/3 -> Gain2/1  "p_dotdot_d"
  Sum9/1 -> Sum6/2  "v_p"
  Gain3/1 -> Sum9/1
  Constant/1 -> Product4/1
  Constant1/1 -> Product4/2
  Derivative6/1 -> Scope/1, Sum1/2
  Constant10/1 -> MATLAB Function12/1(alpha)
  Product16/1 -> Sum1/1
  Constant11/1 -> MATLAB Function12/3(deltah)
  Product17/1 -> Product15/1  "R_BtoI_dotodot"
  MATLAB Function13/1(w_x) -> Product16/1, Derivative6/1, Product16/2
  R_BtoI/1 -> Zero-Order Hold5/1  "R_BtoI"
  Sum1/1 -> Product17/1
  Product4/1 -> Sum6/3
  Gain2/1 -> Sum9/3
  Constant2/1 -> MATLAB Function12/2(beta)
  Constant5/1 -> MATLAB Function12/4(l)
  MATLAB Function12/1(result) -> Gain/1
  Gain/1 -> Product15/2
  Mux2/1 -> u/1
  v_I/1 -> Zero-Order Hold1/1
  "p_d, p_dot_d, p_dotdot_d"/1 -> Zero-Order Hold3/1
  Zero-Order Hold2/1 -> Sum11/1
  Zero-Order Hold1/1 -> Sum10/1
  Zero-Order Hold3/1 -> Demux3/1
  Zero-Order Hold4/1 -> MATLAB Function1/1(R)
  Zero-Order Hold5/1 -> Product17/2, MATLAB Function7/1(R)
  Zero-Order Hold6/1 -> Demux1/1
  Zero-Order Hold7/1 -> MATLAB Function13/1(omega), MATLAB Function11/8(omega_B), Sum3/2

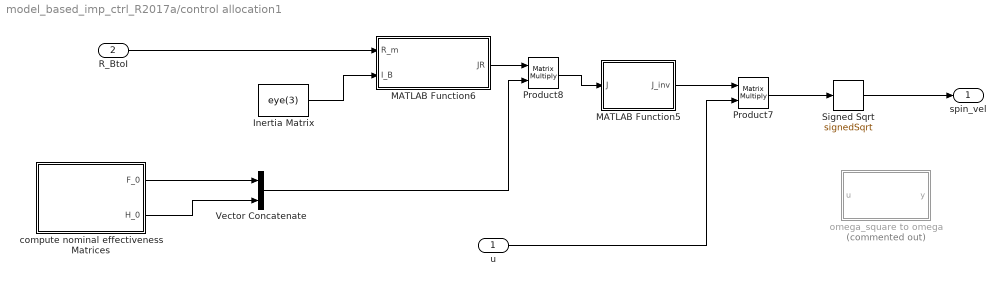
== system model_based_imp_ctrl_R2017a/control allocation1 ==
  u : Inport
  R_BtoI : Inport  Port=2
  Inertia Matrix : Constant  Value=eye(3)  VectorParams1D=off
  MATLAB Function5 : MATLAB Function  TreatAsAtomicUnit=on  SystemSampleTime=Ts
  MATLAB Function6 : MATLAB Function  TreatAsAtomicUnit=on
  Product7 : Product  Multiplication=Matrix(*)
  Product8 : Product  Multiplication=Matrix(*)
  Signed Sqrt : Sqrt  Operator=signedSqrt  SaturateOnIntegerOverflow=on
  Vector Concatenate : Concatenate  Mode=Multidimensional array
  compute nominal effectiveness Matrices : Subsystem
  omega_square to omega : MATLAB Function  Commented=on  TreatAsAtomicUnit=on  SystemSampleTime=Ts
  spin_vel : Outport
  wires:
  MATLAB Function5/1(J_inv) -> Product7/1
  R_BtoI/1 -> MATLAB Function6/1(R_m)
  MATLAB Function6/1(JR) -> Product8/1
  u/1 -> Product7/2
  Inertia Matrix/1 -> MATLAB Function6/2(I_B)
  compute nominal effectiveness Matrices/1(F_0) -> Vector Concatenate/1
  compute nominal effectiveness Matrices/2("H_0 ") -> Vector Concatenate/2
  Product7/1 -> Signed Sqrt/1
  Signed Sqrt/1 -> spin_vel/1
  Vector Concatenate/1 -> Product8/2
  Product8/1 -> MATLAB Function5/1(J)

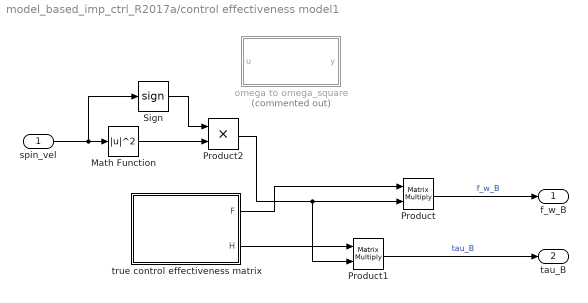
== system model_based_imp_ctrl_R2017a/control effectiveness model1 ==
  spin_vel : Inport
  Math Function : Math  Operator=magnitude^2  SaturateOnIntegerOverflow=on
  Product : Product  Multiplication=Matrix(*)
  Product1 : Product  Multiplication=Matrix(*)
  Product2 : Product
  Sign : Signum
  omega to omega_square : MATLAB Function  Commented=on  TreatAsAtomicUnit=on
  true control effectiveness matrix : Subsystem
  f_w_B : Outport
  tau_B : Outport  Port=2
  wires:
  Product/1 -> f_w_B/1  "f_w_B"
  Product1/1 -> tau_B/1  "tau_B"
  true control effectiveness matrix/1(F) -> Product/1
  true control effectiveness matrix/2(H) -> Product1/1
  spin_vel/1 -> Sign/1, Math Function/1
  Math Function/1 -> Product2/2
  Sign/1 -> Product2/1
  Product2/1 -> Product1/2, Product/2

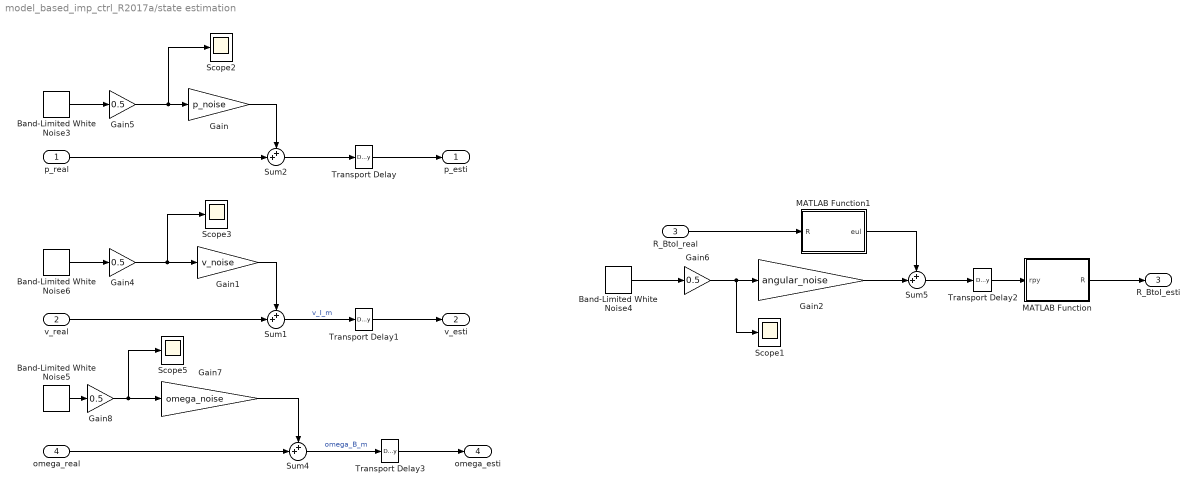
== system model_based_imp_ctrl_R2017a/state estimation ==
  p_real : Inport
  v_real : Inport  Port=2
  R_BtoI_real : Inport  Port=3
  omega_real : Inport  Port=4
  Band-Limited White Noise3 : simulink/Sources/Band-Limited White Noise  Cov=[0.01; 0.01; 0.01]  Ts=Ts  seed=[22352; 29655; 12541]  VectorParams1D=off
  Band-Limited White Noise4 : simulink/Sources/Band-Limited White Noise  Cov=[0.01; 0.01; 0.01]  Ts=Ts  seed=[11351; 22653; 52546]  VectorParams1D=off
  Band-Limited White Noise5 : simulink/Sources/Band-Limited White Noise  Cov=[0.01; 0.01; 0.01]  Ts=Ts  seed=[12451; 82653; 82546]  VectorParams1D=off
  Band-Limited White Noise6 : simulink/Sources/Band-Limited White Noise  Cov=[0.01; 0.01; 0.01]  Ts=Ts  seed=[22351; 29653; 12546]  VectorParams1D=off
  Gain : Gain  Gain=p_noise
  Gain1 : Gain  Gain=v_noise
  Gain2 : Gain  Gain=angular_noise
  Gain{4..6,8} (4 alike) : Gain  Gain=0.5
  Gain7 : Gain  Gain=omega_noise
  MATLAB Function : MATLAB Function  TreatAsAtomicUnit=on
  MATLAB Function1 : MATLAB Function  TreatAsAtomicUnit=on
  Scope{1..3,5} (4 alike) : Scope
  Sum{1..2,4..5} (4 alike) : Sum  Inputs=++|
  Transport Delay{,1..3} (4 alike) : TransportDelay  DelayTime=T_delay  InitialOutput=[0;0;0]
  p_esti : Outport
  v_esti : Outport  Port=2
  R_BtoI_esti : Outport  Port=3
  omega_esti : Outport  Port=4
  wires:
  R_BtoI_real/1 -> MATLAB Function1/1(R)
  p_real/1 -> Sum2/2
  Transport Delay/1 -> p_esti/1
  Sum4/1 -> Transport Delay3/1  "omega_B_m"
  Gain/1 -> Sum2/1
  Gain1/1 -> Sum1/1
  Sum2/1 -> Transport Delay/1
  Sum1/1 -> Transport Delay1/1  "v_I_m"
  MATLAB Function1/1(eul) -> Sum5/1
  Sum5/1 -> Transport Delay2/1
  Gain2/1 -> Sum5/2
  Transport Delay2/1 -> MATLAB Function/1(rpy)
  v_real/1 -> Sum1/2
  omega_real/1 -> Sum4/2
  MATLAB Function/1(R) -> R_BtoI_esti/1
  Transport Delay1/1 -> v_esti/1
  Gain5/1 -> Scope2/1, Gain/1
  Band-Limited White Noise3/1 -> Gain5/1
  Gain4/1 -> Gain1/1, Scope3/1
  Band-Limited White Noise6/1 -> Gain4/1
  Band-Limited White Noise5/1 -> Gain8/1
  Gain8/1 -> Scope5/1, Gain7/1
  Gain6/1 -> Scope1/1, Gain2/1
  Band-Limited White Noise4/1 -> Gain6/1
  Transport Delay3/1 -> omega_esti/1
  Gain7/1 -> Sum4/1

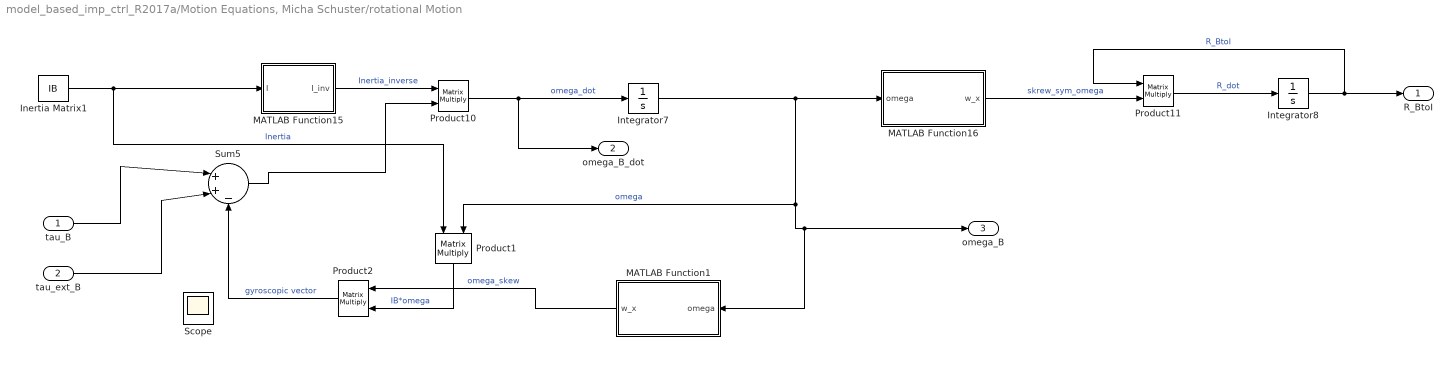
== system model_based_imp_ctrl_R2017a/Motion Equations, Micha Schuster/rotational Motion ==
  tau_B : Inport
  tau_ext_B : Inport  Port=2
  Inertia Matrix1 : Constant  Value=IB  VectorParams1D=off
  Integrator7 : Integrator  InitialCondition=[0 0 0]'
  Integrator8 : Integrator  InitialCondition=[1 0 0; 0 1 0; 0 0 1]
  MATLAB Function1 : MATLAB Function  TreatAsAtomicUnit=on
  MATLAB Function15 : MATLAB Function  TreatAsAtomicUnit=on
  MATLAB Function16 : MATLAB Function  TreatAsAtomicUnit=on
  Product{1..2,10..11} (4 alike) : Product  Multiplication=Matrix(*)
  Scope : Scope
  Sum5 : Sum  Inputs=|++-
  R_BtoI : Outport
  omega_B_dot : Outport  Port=2
  omega_B : Outport  Port=3
  wires:
  Product10/1 -> omega_B_dot/1, Integrator7/1  "omega_dot"
  tau_B/1 -> Sum5/1
  Integrator7/1 -> Product1/2, omega_B/1, MATLAB Function1/1(omega), MATLAB Function16/1(omega)  "omega"
  tau_ext_B/1 -> Sum5/2
  Inertia Matrix1/1 -> Product1/1, MATLAB Function15/1(I)  "Inertia"
  Sum5/1 -> Product10/2
  Product11/1 -> Integrator8/1  "R_dot"
  MATLAB Function15/1(I_inv) -> Product10/1  "Inertia_inverse"
  Integrator8/1 -> Product11/1, R_BtoI/1  "R_BtoI"
  Product2/1 -> Sum5/3  "gyroscopic vector"
  MATLAB Function1/1(w_x) -> Product2/1  "omega_skew"
  Product1/1 -> Product2/2  "IB*omega"
  MATLAB Function16/1(w_x) -> Product11/2  "skrew_sym_omega"

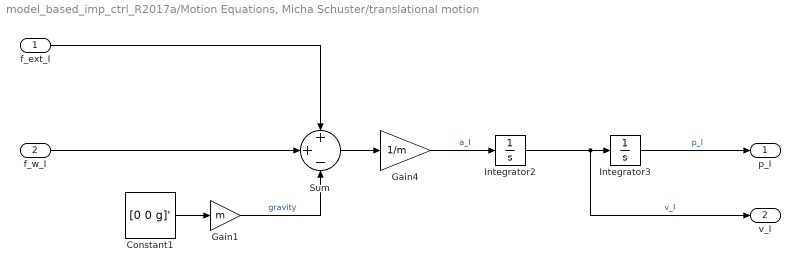
== system model_based_imp_ctrl_R2017a/Motion Equations, Micha Schuster/translational motion ==
  f_ext_I : Inport
  f_w_I : Inport  Port=2
  Constant1 : Constant  Value=[0 0 g]'  VectorParams1D=off
  Gain1 : Gain  Gain=m
  Gain4 : Gain  Gain=1/m
  Integrator2 : Integrator  InitialCondition=[0;0;0]
  Integrator3 : Integrator  InitialCondition=[0 0 0]'
  Sum : Sum  Inputs=++-
  p_I : Outport
  v_I : Outport  Port=2
  wires:
  Sum/1 -> Gain4/1
  f_ext_I/1 -> Sum/1
  Gain4/1 -> Integrator2/1  "a_I"
  Integrator2/1 -> v_I/1, Integrator3/1  "v_I"
  Gain1/1 -> Sum/3  "gravity"
  Constant1/1 -> Gain1/1
  Integrator3/1 -> p_I/1  "p_I"
  f_w_I/1 -> Sum/2

== system model_based_imp_ctrl_R2017a/control allocation1/compute nominal effectiveness Matrices ==
  Constant : Constant  Value=alpha_0
  Constant2 : Constant  Value=beta_0
  Constant3 : Constant  Value=k_0
  Constant4 : Constant  Value=L_0
  Constant5 : Constant  Value=b_0
  MATLAB Function5 : MATLAB Function  TreatAsAtomicUnit=on
  MATLAB Function6 : MATLAB Function  TreatAsAtomicUnit=on
  F_0 : Outport
  "H_0 " : Outport  Port=2
  wires:
  MATLAB Function6/1(F) -> F_0/1
  MATLAB Function6/2(H) -> "H_0 "/1
  Constant5/1 -> MATLAB Function6/7(b)
  Constant/1 -> MATLAB Function5/1(alpha)
  Constant2/1 -> MATLAB Function5/2(beta)
  Constant3/1 -> MATLAB Function6/8(k)
  MATLAB Function5/5(e_r5) -> MATLAB Function6/5(e_r5)
  MATLAB Function5/1(e_r1) -> MATLAB Function6/1(e_r1)
  MATLAB Function5/4(e_r4) -> MATLAB Function6/4(e_r4)
  MATLAB Function5/3(e_r3) -> MATLAB Function6/3(e_r3)
  MATLAB Function5/2(e_r2) -> MATLAB Function6/2(e_r2)
  Constant4/1 -> MATLAB Function6/9(L)
  MATLAB Function5/6(e_r6) -> MATLAB Function6/6(e_r6)

== system model_based_imp_ctrl_R2017a/control effectiveness model1/true control effectiveness matrix ==
  Constant : Constant  Value=alpha
  Constant2 : Constant  Value=beta
  Constant3 : Constant  Value=k
  Constant4 : Constant  Value=L
  Constant5 : Constant  Value=b
  MATLAB Function5 : MATLAB Function  TreatAsAtomicUnit=on
  MATLAB Function6 : MATLAB Function  TreatAsAtomicUnit=on
  F : Outport
  H : Outport  Port=2
  wires:
  MATLAB Function5/6(e_r6) -> MATLAB Function6/6(e_r6)
  Constant4/1 -> MATLAB Function6/9(L)
  MATLAB Function5/2(e_r2) -> MATLAB Function6/2(e_r2)
  MATLAB Function5/3(e_r3) -> MATLAB Function6/3(e_r3)
  MATLAB Function5/4(e_r4) -> MATLAB Function6/4(e_r4)
  MATLAB Function5/1(e_r1) -> MATLAB Function6/1(e_r1)
  MATLAB Function5/5(e_r5) -> MATLAB Function6/5(e_r5)
  Constant3/1 -> MATLAB Function6/8(k)
  Constant2/1 -> MATLAB Function5/2(beta)
  Constant/1 -> MATLAB Function5/1(alpha)
  Constant5/1 -> MATLAB Function6/7(b)
  MATLAB Function6/2(H) -> H/1
  MATLAB Function6/1(F) -> F/1

== matlab function Motion Equations, p_I3/MATLAB Function3 ==
  data: result output double; alpha input double; beta input double; deltah input double; l input double
function result = sum_prop_pos(alpha,beta,deltah,l)

% pi_in_B = zeros(3,6);
result=zeros(3,1);
for it = 1:6
%     alpha_i = alpha *(-1)^(it+1);
    gamma_i = (2*it-3)*pi/6;
    ca = cos(alpha(it));
    sa = sin(alpha(it));
    cb = cos(beta(it));
    sb = sin(beta(it));
    cy = cos(gamma_i);
    sy = sin(gamma_i);
    
%     pi_in_B(:,it) = [deltah*(ca*sb*cy + sa*sy) + l*cy;
%                  deltah*(ca*sb*sy - sa*cy) + l*sy;
%                  deltah*ca*cb];
%     
%     result=result+ pi_in_B(:,it);      

    result = result + [ deltah*(ca*sb*cy + sa*sy) + l*cy;...
                        deltah*(ca*sb*sy - sa*cy) + l*sy;...
                        deltah*ca*cb];...
end

== matlab function Motion Equations, p_I3/MATLAB Function1 ==
  data: omega input double; w_x output double
function w_x = omegaSkew3D(omega)

w_x = [0 -omega(3) omega(2);
        omega(3) 0 -omega(1);
        -omega(2) omega(1) 0];

== matlab function MATLAB Function4 ==
  data: R input double; eul output double
function eul = DCM2Euler(R)

%Roll
phi = atan2d(R(3,2),R(3,3));

%Pitch
psi = atan2d(-R(3,1),sqrt(R(1,1)^2 + R(2,1)^2));

%Yaw
gamma = atan2d(R(2,1),R(1,1));

eul=[phi;psi;gamma];

== matlab function Motion Equations, Micha Schuster/rotational Motion/MATLAB Function1 ==
  data: omega input double; w_x output double
function w_x = Skew3D(omega)

w_x = [0 -omega(3) omega(2);
        omega(3) 0 -omega(1);
        -omega(2) omega(1) 0];

== matlab function Motion Equations, Micha Schuster/rotational Motion/MATLAB Function15 ==
  data: I input double; I_inv output double
function I_inv = inverse(I)

I_inv = inv(I);

== matlab function Motion Equations, Micha Schuster/rotational Motion/MATLAB Function16 ==
  data: omega input double; w_x output double
function w_x = omegaSkew3D(omega)

w_x = [0 -omega(3) omega(2);
        omega(3) 0 -omega(1);
        -omega(2) omega(1) 0];

== matlab function control allocation1/MATLAB Function5 ==
  data: J input double; J_inv output double
function J_inv = inverse(J)

J_inv = inv(J);

== matlab function control allocation1/MATLAB Function6 ==
  data: R_m input double; JR output double; I_B input double
function JR = computeJR(R_m, I_B)
JR = [R_m zeros(3);
     zeros(3) inv(I_B) ];

== matlab function combination of Imp and slid_Control/MATLAB Function12 ==
  data: result output double; alpha input double; beta input double; deltah input double; l input double
function result = sum_prop_pos(alpha,beta,deltah,l)

% pi_in_B = zeros(3,6);
result=zeros(3,1);
for it = 1:6
%     alpha_i = alpha *(-1)^(it+1);
    gamma_i = (2*it-3)*pi/6;
    ca = cos(alpha(it));
    sa = sin(alpha(it));
    cb = cos(beta(it));
    sb = sin(beta(it));
    cy = cos(gamma_i);
    sy = sin(gamma_i);
    
%     pi_in_B(:,it) = [deltah*(ca*sb*cy + sa*sy) + l*cy;
%                  deltah*(ca*sb*sy - sa*cy) + l*sy;
%                  deltah*ca*cb];
%     
%     result=result+ pi_in_B(:,it);      

    result = result + [ deltah*(ca*sb*cy + sa*sy) + l*cy;...
                        deltah*(ca*sb*sy - sa*cy) + l*sy;...
                        deltah*ca*cb];...
end

== matlab function Trajectory Generator ==
  data: t input double; p_d output double; p_d_dot output double; p_d_dotdot output double; R_d output double; omega_d output double; omega_d_dot output double; T_D output double; T_D_dot output double
function [p_d, p_d_dot, p_d_dotdot, R_d, omega_d, omega_d_dot, T_D, T_D_dot] = createTrajectory(t)

% if t < 1
%     %zeros
%     % 
%     p_d = [0;0;0];
%     p_d_dot = [0;0;0];
%     p_d_dotdot = [0;0;0];
%     R_d = eye(3);
%     omega_d = [0;0;0];
%     omega_d_dot = [0;0;0];
%     T_D = zeros(6,1);
%     T_D_dot = zeros(6,1);
% 
% else
%    % p_d = [1;0.75;0.5];
%     p_d = [0;0;0];
%     p_d_dot = [0;0;0];
%     p_d_dotdot = [0;0;0];
%     
%     ct = cosd(7.5);
%     st = sind(7.5);
%     ct2 = cosd(10);
%     st2 = sind(10);
%     R_d = [ct, 0, st; 
%             0, 1, 0;
%             -st, 0, ct]*[1 0 0;
%             0 ct2, -st2; 
%            0 st2, ct2];
%     omega_d = [0;0;0];
%     omega_d_dot = [0;0;0];
%     T_D = zeros(6,1);
%     T_D_dot = zeros(6,1);
    
%     
%         t = t-10;
%     xa = 0;
%     xe = 1;
%     te = 5;
%     x = xa + 10*(xe-xa)*t^3/te^3 - 15*(xe-xa)*t^4/te^4 + 6*(xe-xa)*t^5/te^5;
%     x_dot = 3*10*(xe-xa)*t^2/te^3 - 4*15*(xe-xa)*t^3/te^4 + 5*6*(xe-xa)*t^4/te^5;
%     x_dot_dot = 6*10*(xe-xa)*t/te^3 - 12*15*(xe-xa)*t^2/te^4 + 20*6*(xe-xa)*t^3/te^5;
%     if (t> te)
%         x = xe;
%         x_dot = 0;
%         x_dot_dot = 0;
%     end
%     p_d = [x;0;x];
%     p_d_dot = [x_dot;0;x_dot];
%     p_d_dotdot = [x_dot_dot;0;x_dot_dot];
%     
%     xe = 0.5;
%     x = xa + 10*(xe-xa)*t^3/te^3 - 15*(xe-xa)*t^4/te^4 + 6*(xe-xa)*t^5/te^5;
%     x_dot = 3*10*(xe-xa)*t^2/te^3 - 4*15*(xe-xa)*t^3/te^4 + 5*6*(xe-xa)*t^4/te^5;
%     x_dot_dot = 6*10*(xe-xa)*t/te^3 - 12*15*(xe-xa)*t^2/te^4 + 20*6*(xe-xa)*t^3/te^5;
%     if (t> te)
%         x = xe;
%         x_dot = 0;
%         x_dot_dot = 0;
%     end
%     p_d(3) = x;
%     p_d_dot(3) = x_dot;
%     p_d_dotdot(3) = x_dot_dot;
%     
%     a = 2*pi/te;
%     ct = cos(a*t);
%     st = sin(a*t);
%     
%     R_d = [ct, -st, 0; 
%            st, ct, 0;
%            0 0 1];
%     R_d_dot = [-a*st, -a*ct, 0;
%                 a*ct, -a*st, 0;
%                 0 0 0];
%     R_d_dotdot = [-a*a*ct, a*a*st, 0;
%                    -a*a*st, -a*a*ct, 0;
%                    0 0 0];
%                
%     T_d_tilde = [R_d', -R_d'*p_d; 0,0,0,1]*[R_d_dot p_d_dot; 0,0,0,0];
%     
%     omega_d = skew2vec(T_d_tilde(1:3,1:3));
%     
%     T_d_tilde_dot = [R_d_dot'*R_d_dot+R_d'*R_d_dotdot, R_d_dot'*p_d_dot+R_d'*p_d_dotdot;
%         0,0,0,0];
%     
%     omega_d_dot = skew2vec(T_d_tilde_dot(1:3,1:3));
%     
%     T_D = [omega_d; T_d_tilde(1:3,4)];
%     T_D_dot = [omega_d_dot; T_d_tilde_dot(1:3,4)];
%     
%     if t>te
%         R_d = eye(3);
%         omega_d = [0;0;0];
%         omega_d_dot = [0;0;0];
%         T_D = zeros(6,1);
%         T_D_dot = zeros(6,1);
%     end
% end
% 
    p_d = [0;0;0];
    p_d_dot = [0;0;0];
    p_d_dotdot = [0;0;0];
    R_d = eye(3);
    omega_d = [0;0;0];
    omega_d_dot = [0;0;0];
    T_D = zeros(6,1);
    T_D_dot = zeros(6,1);

== matlab function combination of Imp and slid_Control/MATLAB Function13 ==
  data: omega input double; w_x output double
function w_x = omegaSkew3D(omega)

w_x = [0 -omega(3) omega(2);
        omega(3) 0 -omega(1);
        -omega(2) omega(1) 0];
